simulink model "eeg8_demo"  (R2018a)
settings: Solver=VariableStepAuto  StartTime=0.0  StopTime=inf  RelTol=1e-3
undefined symbols (not defined in the file or in its folder): fdesignblkfcn, gcbh
libraries: dspindex x1
(part 2 of 5)

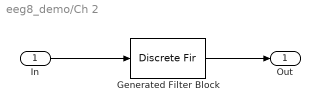
== system eeg8_demo/Ch 2 ==
  In : Inport
  Generated Filter Block : DiscreteFir  Tag=BlockMethodSubSystem  Coefficients=[-0.0012057604808034415 -0.00400942881040558009 -0.00626561744168136359 -0.00738801392416177719 -0.00527276815990392923 -0.000919338487558358499 0.00368732452081514846 0.00579877927647547402 0.00462402170615156243 0.00158437513563851849 -0.000633672902673079025 -0.000429755197249887953 0.00157474318304429736 0.00325954236691781843 0.00306882343350810098 0.0013523573892122063 -0.000139868198508621701 -5.70581879558289487e-05 0.00129014205749712553 0.00237886387142490548 0.00208573560494999767 0.000775896474187955814 -0.000181711655680853561 0.000115848037873191582 0.00121090357790058778 0.00185271800445839388 0.00135326703938135344 0.000270939254141498525 -0.000253835419574898748 0.000259733798241630566 0.00115808320311440081 0.00141449499387325981 0.000750062990649251666 -0.000105171655205074996 -0.0002493465299276854 0.000404856115638034942 0.00107161023472011874 0.000988284588860301313 0.000248113916671139874 -0.000336862076385113459 -0.00015659378164813162 0.000531318192704894167 0.000918767983170676837 0.000560650407515253524 -0.000144207271933711453 -0.000423105433409615768 -2.4157603152224956e-06 0.000602893137126713267 0.000687619992885029393 0.000149865361744685695 -0.000409682086252503863 -0.000381262084932819725 0.00016841365431926678 0.000588220835854016836 0.000388593216913443653 -0.000208577391166257228 -0.000536149531578196587 -0.000245643601967410739 0.000305369347432664395 0.000470503838642328317 5.38522428589523753e-05 -0.000475790002075137069 -0.000528485587882095847 -6.56127452976172632e-05 0.000363387906024332553 0.00025622248435134301 -0.000270954870593259004 -0.000623482691174682122 -0.000412760429073543702 0.000101066425823716251 0.000314676982032867575 -2.57132385341216229e-05 -0.000536045338262289999 -0.000640676976997142655 -0.000234132718753334371 0.000202379083484820519 0.000156243345085702203 -0.00032659743096525402 -0.000698706059465434531 -0.000542770108742592766 -5.04551108064955884e-05 0.000200058711149488365 -8.81624465044778281e-05 -0.000590876422546488087 -0.000737059879079341959 -0.00036835435804223165 8.01517605901424889e-05 8.21955409095078397e-05 -0.00037261663135342997 -0.000766946333356812219 -0.000654143076503351981 -0.00017252064049063802 0.00011328273030307297 -0.000134772344149603851 -0.000637991962663725398 -0.000822622491623204127 -0.000481974408500684536 -1.68008834177117133e-05 2.81525576195080065e-05 -0.000407364672766683574 -0.000827241362232989308 -0.000752485508647688533 -0.000274559803509483082 4.78470606035301808e-05 -0.000165436317645622295 -0.000675561930527132106 -0.000898942926045737827 -0.000581224292971747316 -9.40989017609547866e-05 -6.57962314188595459e-06 -0.0004277474404043796 -0.00087702323616187434 -0.000839009094129124894 -0.000359936983533792594 2.4697782641331057e-06 -0.000177397096814225781 -0.00069843510903147229 -0.000962901883298498745 -0.000666342952086573315 -0.000153400772580388189 -2.13240775285701975e-05 -0.000430018204075204925 -0.000912330950373263201 -0.000913073764468091292 -0.000430660819379980993 -2.46801764465285248e-05 -0.000168776382482316745 -0.000702089423485303824 -0.00100968908285008186 -0.000733920595496317181 -0.000190950202251182171 -1.00121307305317941e-05 -0.000405238623582842357 -0.000924319752905339363 -0.000967624947644758174 -0.000483359168684824563 -3.17683843657163634e-05 -0.000139569941291287894 -0.000687509099616782698 -0.0010427176195738244 -0.000789077389326541608 -0.000212236046414509286 2.48347794344122217e-05 -0.000351879253188750656 -0.000907069288605061438 -0.000994920529897785856 -0.000507833293495327937 -5.46833481983312383e-06 -7.07610372629760933e-05 -0.00063207754920801358 -0.0010398946657567314 -0.000815391687157836979 -0.000208829247240500563 8.38928391407327734e-05 -0.000275785916268746277 -0.000872071258521420721 -0.00101095317444154062 -0.000522573473808359544 3.62427877631585208e-05 2.26702521635803859e-05 -0.000546410627995994936 -0.00100739237485209486 -0.000815055820324720446 -0.000177872322615011102 ...(+20136 chars)]  InputProcessing=Columns as channels (frame based)
  Out : Outport
  wires:
  In/1 -> Generated Filter Block/1
  Generated Filter Block/1 -> Out/1

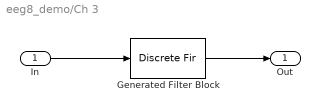
== system eeg8_demo/Ch 3 ==
  In : Inport
  Generated Filter Block : DiscreteFir  Tag=BlockMethodSubSystem  Coefficients=[-0.0012057604808034415 -0.00400942881040558009 -0.00626561744168136359 -0.00738801392416177719 -0.00527276815990392923 -0.000919338487558358499 0.00368732452081514846 0.00579877927647547402 0.00462402170615156243 0.00158437513563851849 -0.000633672902673079025 -0.000429755197249887953 0.00157474318304429736 0.00325954236691781843 0.00306882343350810098 0.0013523573892122063 -0.000139868198508621701 -5.70581879558289487e-05 0.00129014205749712553 0.00237886387142490548 0.00208573560494999767 0.000775896474187955814 -0.000181711655680853561 0.000115848037873191582 0.00121090357790058778 0.00185271800445839388 0.00135326703938135344 0.000270939254141498525 -0.000253835419574898748 0.000259733798241630566 0.00115808320311440081 0.00141449499387325981 0.000750062990649251666 -0.000105171655205074996 -0.0002493465299276854 0.000404856115638034942 0.00107161023472011874 0.000988284588860301313 0.000248113916671139874 -0.000336862076385113459 -0.00015659378164813162 0.000531318192704894167 0.000918767983170676837 0.000560650407515253524 -0.000144207271933711453 -0.000423105433409615768 -2.4157603152224956e-06 0.000602893137126713267 0.000687619992885029393 0.000149865361744685695 -0.000409682086252503863 -0.000381262084932819725 0.00016841365431926678 0.000588220835854016836 0.000388593216913443653 -0.000208577391166257228 -0.000536149531578196587 -0.000245643601967410739 0.000305369347432664395 0.000470503838642328317 5.38522428589523753e-05 -0.000475790002075137069 -0.000528485587882095847 -6.56127452976172632e-05 0.000363387906024332553 0.00025622248435134301 -0.000270954870593259004 -0.000623482691174682122 -0.000412760429073543702 0.000101066425823716251 0.000314676982032867575 -2.57132385341216229e-05 -0.000536045338262289999 -0.000640676976997142655 -0.000234132718753334371 0.000202379083484820519 0.000156243345085702203 -0.00032659743096525402 -0.000698706059465434531 -0.000542770108742592766 -5.04551108064955884e-05 0.000200058711149488365 -8.81624465044778281e-05 -0.000590876422546488087 -0.000737059879079341959 -0.00036835435804223165 8.01517605901424889e-05 8.21955409095078397e-05 -0.00037261663135342997 -0.000766946333356812219 -0.000654143076503351981 -0.00017252064049063802 0.00011328273030307297 -0.000134772344149603851 -0.000637991962663725398 -0.000822622491623204127 -0.000481974408500684536 -1.68008834177117133e-05 2.81525576195080065e-05 -0.000407364672766683574 -0.000827241362232989308 -0.000752485508647688533 -0.000274559803509483082 4.78470606035301808e-05 -0.000165436317645622295 -0.000675561930527132106 -0.000898942926045737827 -0.000581224292971747316 -9.40989017609547866e-05 -6.57962314188595459e-06 -0.0004277474404043796 -0.00087702323616187434 -0.000839009094129124894 -0.000359936983533792594 2.4697782641331057e-06 -0.000177397096814225781 -0.00069843510903147229 -0.000962901883298498745 -0.000666342952086573315 -0.000153400772580388189 -2.13240775285701975e-05 -0.000430018204075204925 -0.000912330950373263201 -0.000913073764468091292 -0.000430660819379980993 -2.46801764465285248e-05 -0.000168776382482316745 -0.000702089423485303824 -0.00100968908285008186 -0.000733920595496317181 -0.000190950202251182171 -1.00121307305317941e-05 -0.000405238623582842357 -0.000924319752905339363 -0.000967624947644758174 -0.000483359168684824563 -3.17683843657163634e-05 -0.000139569941291287894 -0.000687509099616782698 -0.0010427176195738244 -0.000789077389326541608 -0.000212236046414509286 2.48347794344122217e-05 -0.000351879253188750656 -0.000907069288605061438 -0.000994920529897785856 -0.000507833293495327937 -5.46833481983312383e-06 -7.07610372629760933e-05 -0.00063207754920801358 -0.0010398946657567314 -0.000815391687157836979 -0.000208829247240500563 8.38928391407327734e-05 -0.000275785916268746277 -0.000872071258521420721 -0.00101095317444154062 -0.000522573473808359544 3.62427877631585208e-05 2.26702521635803859e-05 -0.000546410627995994936 -0.00100739237485209486 -0.000815055820324720446 -0.000177872322615011102 ...(+20136 chars)]  InputProcessing=Columns as channels (frame based)
  Out : Outport
  wires:
  In/1 -> Generated Filter Block/1
  Generated Filter Block/1 -> Out/1
